simulink model "SecRwLtStCalib"  (R2024b)
settings: Solver=FixedStepDiscrete  StartTime=0.0  StopTime=10.0  FixedStep=0.01  RelTol=1e-3
model workspace (MAT data in the model file):
  KeSMSwAcsMd6SecRwLtStBkReclnUpwdDnwdPos1Max_Val : Simulink.Parameter (value not decoded)
  KeSMSwAcsMd6SecRwLtStBkReclnUpwdDnwdPos1Min_Val : Simulink.Parameter (value not decoded)
  KeSMSwAcsMd6SecRwLtStBkReclnUpwdDnwdPos1_Val : Simulink.Parameter (value not decoded)
  KeSMSwAcsMd6SecRwLtStBkReclnUpwdDnwdPosMax_Val : Simulink.Parameter (value not decoded)
  KeSMSwAcsMd6SecRwLtStBkReclnUpwdDnwdPosMin_Val : Simulink.Parameter (value not decoded)
  KeSMSwAcsMd6SecRwLtStBkReclnUpwdDnwdPos_Val : Simulink.Parameter (value not decoded)
symbols that are objects in the model workspace (value not decoded): KeSMSwAcsMd6SecRwLtStBkReclnUpwdDnwdPos1_Val, KeSMSwAcsMd6SecRwLtStBkReclnUpwdDnwdPos1Max_Val, KeSMSwAcsMd6SecRwLtStBkReclnUpwdDnwdPos1Min_Val, KeSMSwAcsMd6SecRwLtStBkReclnUpwdDnwdPos_Val, KeSMSwAcsMd6SecRwLtStBkReclnUpwdDnwdPosMax_Val, KeSMSwAcsMd6SecRwLtStBkReclnUpwdDnwdPosMin_Val
undefined symbols (not defined in the file or in its folder): KeSMSw4SAcsMd21SecRwLtStBkReclnUpwdDnwdPos_Val, KeSMSw4SAcsMd21SecRwLtStBkReclnUpwdDnwdPosMax_Val, KeSMSw4SAcsMd21SecRwLtStBkReclnUpwdDnwdPosMin_Val, KeSMSw4SAcsMd21SecRwLtStFrwdBkwdPos_Val, KeSMSw4SAcsMd21SecRwLtStFrwdBkwdPosMax_Val, KeSMSw4SAcsMd21SecRwLtStFrwdBkwdPosMin_Val, KeSMSw4SAcsMd21SecRwLtStHdrstFrwdBkwdPos_Val, KeSMSw4SAcsMd21SecRwLtStHdrstFrwdBkwdPosMax_Val, KeSMSw4SAcsMd21SecRwLtStHdrstFrwdBkwdPosMin_Val, KeSMSw4SAcsMd21SecRwLtStHdrstUpwdDnwdPos_Val, KeSMSw4SAcsMd21SecRwLtStHdrstUpwdDnwdPosMax_Val, KeSMSw4SAcsMd21SecRwLtStHdrstUpwdDnwdPosMin_Val, KeSMSw4SAcsMd22SecRwLtStBkReclnUpwdDnwdPos1_Val, KeSMSw4SAcsMd22SecRwLtStBkReclnUpwdDnwdPos2_Val, KeSMSw4SAcsMd22SecRwLtStBkReclnUpwdDnwdPos2Max_Val, KeSMSw4SAcsMd22SecRwLtStBkReclnUpwdDnwdPos2Min_Val, KeSMSw4SAcsMd22SecRwLtStBkReclnUpwdDnwdPosMax_Val, KeSMSw4SAcsMd22SecRwLtStBkReclnUpwdDnwdPosMin_Val, KeSMSw4SAcsMd22SecRwLtStFrwdBkwdPos_Val, KeSMSw4SAcsMd22SecRwLtStFrwdBkwdPosMax_Val, KeSMSw4SAcsMd22SecRwLtStFrwdBkwdPosMin_Val, KeSMSw4SAcsMd22SecRwLtStFtrstUpwdDnwdPos_Val, KeSMSw4SAcsMd22SecRwLtStFtrstUpwdDnwdPosMax_Val, KeSMSw4SAcsMd22SecRwLtStFtrstUpwdDnwdPosMin_Val, KeSMSw4SAcsMd22SecRwLtStHdrstFrwdBkwdPos_Val, KeSMSw4SAcsMd22SecRwLtStHdrstFrwdBkwdPosMax_Val, KeSMSw4SAcsMd22SecRwLtStHdrstFrwdBkwdPosMin_Val, KeSMSw4SAcsMd22SecRwLtStHdrstUpwdDnwdPos_Val, KeSMSw4SAcsMd22SecRwLtStHdrstUpwdDnwdPosMax_Val, KeSMSw4SAcsMd22SecRwLtStHdrstUpwdDnwdPosMin_Val, KeSMSw4SAcsMd22SecRwLtStLegrstOtwdInwdPos_Val, KeSMSw4SAcsMd22SecRwLtStLegrstOtwdInwdPosMax_Val, KeSMSw4SAcsMd22SecRwLtStLegrstOtwdInwdPosMin_Val, KeSMSw4SAcsMd22SecRwLtStLegrstUpwdDnwdPos_Val, KeSMSw4SAcsMd22SecRwLtStLegrstUpwdDnwdPosMax_Val, KeSMSw4SAcsMd22SecRwLtStLegrstUpwdDnwdPosMin_Val, KeSMSw4SAcsMd25SecRwLtStBkReclnUpwdDnwdPos_Val, KeSMSw4SAcsMd25SecRwLtStBkReclnUpwdDnwdPosMax_Val, KeSMSw4SAcsMd25SecRwLtStBkReclnUpwdDnwdPosMin_Val, KeSMSw4SAcsMd25SecRwLtStFrwdBkwdPos_Val, KeSMSw4SAcsMd25SecRwLtStFrwdBkwdPosMax_Val, KeSMSw4SAcsMd25SecRwLtStFrwdBkwdPosMin_Val, KeSMSw4SAcsMd25SecRwLtStHdrstFrwdBkwdPos_Val, KeSMSw4SAcsMd25SecRwLtStHdrstFrwdBkwdPosMax_Val, KeSMSw4SAcsMd25SecRwLtStHdrstFrwdBkwdPosMin_Val, KeSMSw4SAcsMd25SecRwLtStHdrstUpwdDnwdPos_Val, KeSMSw4SAcsMd25SecRwLtStHdrstUpwdDnwdPosMax_Val, KeSMSw4SAcsMd25SecRwLtStHdrstUpwdDnwdPosMin_Val, KeSMSw4SAcsMd26SecRwLtStBkReclnUpwdDnwdPos_Val, KeSMSw4SAcsMd26SecRwLtStBkReclnUpwdDnwdPosMax_Val, KeSMSw4SAcsMd26SecRwLtStBkReclnUpwdDnwdPosMin_Val, KeSMSw4SAcsMd26SecRwLtStFrwdBkwdPos_Val, KeSMSw4SAcsMd26SecRwLtStFrwdBkwdPosMax_Val, KeSMSw4SAcsMd26SecRwLtStFrwdBkwdPosMin_Val, KeSMSw4SAcsMd26SecRwLtStFtrstUpwdDnwdPos_Val, KeSMSw4SAcsMd26SecRwLtStFtrstUpwdDnwdPosMax_Val, KeSMSw4SAcsMd26SecRwLtStFtrstUpwdDnwdPosMin_Val, KeSMSw4SAcsMd26SecRwLtStHdrstFrwdBkwdPos_Val, KeSMSw4SAcsMd26SecRwLtStHdrstFrwdBkwdPosMax_Val, KeSMSw4SAcsMd26SecRwLtStHdrstFrwdBkwdPosMin_Val ... (+496)
libraries: TrgtPosSelcLib x61, StIsPosChkLib x1, simulink x1
(part 7 of 8)

== system SecRwLtStCalib/SecRwLtStLgrstInwdOtwdTrgtPosSelc_1_Cal_sys/Subsystem2/Subsystem ==
  note: 2023.8.1 V2.0.0 CR401790 增加模式21-26
  StNumFlg_Is6s_read : Inport
  Enable : EnablePort
  Constant : Constant  Value=4095  OutDataTypeStr=uint16
  Constant1 : Constant  Value=4095  OutDataTypeStr=uint16
  Constant2 : Constant  Value=4095  OutDataTypeStr=uint16
  Data Type Conversion{,1..6} (7 alike) : DataTypeConversion  SaturateOnIntegerOverflow=off  RndMeth=Floor
  PA_KeSMSw4SAcsMd22SecRwLtStLegrstOtwdInwdPosMax_Val : Constant  Value=KeSMSw4SAcsMd22SecRwLtStLegrstOtwdInwdPosMax_Val
  PA_KeSMSw4SAcsMd22SecRwLtStLegrstOtwdInwdPosMin_Val : Constant  Value=KeSMSw4SAcsMd22SecRwLtStLegrstOtwdInwdPosMin_Val
  PA_KeSMSw4SAcsMd22SecRwLtStLegrstOtwdInwdPos_Val : Constant  Value=KeSMSw4SAcsMd22SecRwLtStLegrstOtwdInwdPos_Val
  PA_KeSMSw4SAcsMd26SecRwLtStLegrstOtwdInwdPosMax_Val : Constant  Value=KeSMSw4SAcsMd26SecRwLtStLegrstOtwdInwdPosMax_Val
  PA_KeSMSw4SAcsMd26SecRwLtStLegrstOtwdInwdPosMin_Val : Constant  Value=KeSMSw4SAcsMd26SecRwLtStLegrstOtwdInwdPosMin_Val
  PA_KeSMSw4SAcsMd26SecRwLtStLegrstOtwdInwdPos_Val : Constant  Value=KeSMSw4SAcsMd26SecRwLtStLegrstOtwdInwdPos_Val
  PA_KeSMSw4SLegrstCloseMdSecRwLtStLgrstOtwdInwdPosMax_Val : Constant  Value=KeSMSw4SLegrstCloseMdSecRwLtStLgrstOtwdInwdPosMax_Val
  PA_KeSMSw4SLegrstCloseMdSecRwLtStLgrstOtwdInwdPosMin_Val : Constant  Value=KeSMSw4SLegrstCloseMdSecRwLtStLgrstOtwdInwdPosMin_Val
  PA_KeSMSw4SLegrstCloseMdSecRwLtStLgrstOtwdInwdPos_Val : Constant  Value=KeSMSw4SLegrstCloseMdSecRwLtStLgrstOtwdInwdPos_Val
  PA_KeSMSw4SLegrstOpenMdSecRwLtStLgrstOtwdInwdPosMax_Val : Constant  Value=KeSMSw4SLegrstOpenMdSecRwLtStLgrstOtwdInwdPosMax_Val
  PA_KeSMSw4SLegrstOpenMdSecRwLtStLgrstOtwdInwdPosMin_Val : Constant  Value=KeSMSw4SLegrstOpenMdSecRwLtStLgrstOtwdInwdPosMin_Val
  PA_KeSMSw4SLegrstOpenMdSecRwLtStLgrstOtwdInwdPos_Val : Constant  Value=KeSMSw4SLegrstOpenMdSecRwLtStLgrstOtwdInwdPos_Val
  PA_KeSMSw6SAcsMd56SecRwLtStLgrstInwdOtwdPosMax_Val : Constant  Value=KeSMSw6SAcsMd56SecRwLtStLgrstInwdOtwdPosMax_Val
  PA_KeSMSw6SAcsMd56SecRwLtStLgrstInwdOtwdPosMin_Val : Constant  Value=KeSMSw6SAcsMd56SecRwLtStLgrstInwdOtwdPosMin_Val
  PA_KeSMSw6SAcsMd56SecRwLtStLgrstInwdOtwdPos_Val : Constant  Value=KeSMSw6SAcsMd56SecRwLtStLgrstInwdOtwdPos_Val
  PA_KeSMSw6sAcsEntrySecRwLtStLgrstInwdOtwdPosMax_Val : Constant  Value=KeSMSw6sAcsEntrySecRwLtStLgrstInwdOtwdPosMax_Val
  PA_KeSMSw6sAcsEntrySecRwLtStLgrstInwdOtwdPosMin_Val : Constant  Value=KeSMSw6sAcsEntrySecRwLtStLgrstInwdOtwdPosMin_Val
  PA_KeSMSw6sAcsEntrySecRwLtStLgrstInwdOtwdPos_Val : Constant  Value=KeSMSw6sAcsEntrySecRwLtStLgrstInwdOtwdPos_Val
  PA_KeSMSwAcsEntrySecRwLtStLgrstInwdOtwdPosMax_Val : Constant  Value=KeSMSwAcsEntrySecRwLtStLgrstInwdOtwdPosMax_Val
  PA_KeSMSwAcsEntrySecRwLtStLgrstInwdOtwdPosMin_Val : Constant  Value=KeSMSwAcsEntrySecRwLtStLgrstInwdOtwdPosMin_Val
  PA_KeSMSwAcsEntrySecRwLtStLgrstInwdOtwdPos_Val : Constant  Value=KeSMSwAcsEntrySecRwLtStLgrstInwdOtwdPos_Val
  PA_KeSMSwAcsMd56SecRwLtStLgrstInwdOtwdPosMax_Val : Constant  Value=KeSMSwAcsMd56SecRwLtStLgrstInwdOtwdPosMax_Val
  PA_KeSMSwAcsMd56SecRwLtStLgrstInwdOtwdPosMin_Val : Constant  Value=KeSMSwAcsMd56SecRwLtStLgrstInwdOtwdPosMin_Val
  PA_KeSMSwAcsMd56SecRwLtStLgrstInwdOtwdPos_Val : Constant  Value=KeSMSwAcsMd56SecRwLtStLgrstInwdOtwdPos_Val
  PA_KeSMSwAcsMd8SecRwLtStLgrstInwdOtwdPosMax_Val : Constant  Value=KeSMSwAcsMd8SecRwLtStLgrstInwdOtwdPosMax_Val
  PA_KeSMSwAcsMd8SecRwLtStLgrstInwdOtwdPosMin_Val : Constant  Value=KeSMSwAcsMd8SecRwLtStLgrstInwdOtwdPosMin_Val
  PA_KeSMSwAcsMd8SecRwLtStLgrstInwdOtwdPos_Val : Constant  Value=KeSMSwAcsMd8SecRwLtStLgrstInwdOtwdPos_Val
  TrgtPosSelcNo4sMd : TrgtPosSelcLib/TrgtPosSelcNo4sMd  SystemSampleTime=-1  VariantActivationTime=update diagram  AllowFlexibleInterface=on  Latency=0  AutoFrameSizeCalculation=off
  TrgtPosSelcNo4sMd1 : TrgtPosSelcLib/TrgtPosSelcNo4sMd  SystemSampleTime=-1  VariantActivationTime=update diagram  AllowFlexibleInterface=on  Latency=0  AutoFrameSizeCalculation=off
  TrgtPosSelcNo4sMd2 : TrgtPosSelcLib/TrgtPosSelcNo4sMd  SystemSampleTime=-1  VariantActivationTime=update diagram  AllowFlexibleInterface=on  Latency=0  AutoFrameSizeCalculation=off
  TrgtPosSelcOnly4sMd{,1..3} (4 alike) : TrgtPosSelcLib/TrgtPosSelcOnly4sMd  SystemSampleTime=-1  VariantActivationTime=update diagram  AllowFlexibleInterface=on  Latency=0  AutoFrameSizeCalculation=off
  LgrstCloseLR2LLgrstInwdOtwdTrgtPosCalib_TrgtPosArray_write : Outport  VectorParamsAs1DForOutWhenUnconnected=off
  LgrstOpen4sLR2LLgrstInwdOtwdTrgtPosCalib_TrgtPosArray_write : Outport  Port=2  VectorParamsAs1DForOutWhenUnconnected=off
  KeSMSw4SAcsMd22LgrstInwdOtwdTrgtPosCalib_TrgtPosArray_write : Outport  Port=3  VectorParamsAs1DForOutWhenUnconnected=off
      settings: EnsureOutportIsVirtual=on
  KeSMSw4SAcsMd26LgrstInwdOtwdTrgtPosCalib_TrgtPosArray_write : Outport  Port=4  VectorParamsAs1DForOutWhenUnconnected=off
      settings: EnsureOutportIsVirtual=on
  KeSMSwEZEEntryLgrstInwdOtwdTrgtPosCalib_TrgtPosArray_write : Outport  Port=5  VectorParamsAs1DForOutWhenUnconnected=off
      settings: EnsureOutportIsVirtual=on
  Md56LgrstInwdOtwdTrgtPosCalib_TrgtPosArray_write : Outport  Port=6  VectorParamsAs1DForOutWhenUnconnected=off
      settings: EnsureOutportIsVirtual=on
  Md8R2LLgrstInwdOtwdTrgtPosCalib_TrgtPosArray_write : Outport  Port=7  VectorParamsAs1DForOutWhenUnconnected=off
      settings: EnsureOutportIsVirtual=on
  wires:
  PA_KeSMSw4SLegrstCloseMdSecRwLtStLgrstOtwdInwdPos_Val/1 -> TrgtPosSelcOnly4sMd/1
  TrgtPosSelcOnly4sMd1/1 -> Data Type Conversion1/1
  TrgtPosSelcOnly4sMd/1 -> Data Type Conversion/1
  PA_KeSMSw4SLegrstOpenMdSecRwLtStLgrstOtwdInwdPosMin_Val/1 -> TrgtPosSelcOnly4sMd1/3
  PA_KeSMSw4SLegrstOpenMdSecRwLtStLgrstOtwdInwdPosMax_Val/1 -> TrgtPosSelcOnly4sMd1/2
  PA_KeSMSw4SLegrstCloseMdSecRwLtStLgrstOtwdInwdPosMin_Val/1 -> TrgtPosSelcOnly4sMd/3
  PA_KeSMSw4SLegrstOpenMdSecRwLtStLgrstOtwdInwdPos_Val/1 -> TrgtPosSelcOnly4sMd1/1
  PA_KeSMSw4SLegrstCloseMdSecRwLtStLgrstOtwdInwdPosMax_Val/1 -> TrgtPosSelcOnly4sMd/2
  TrgtPosSelcOnly4sMd2/1 -> Data Type Conversion2/1
  TrgtPosSelcOnly4sMd3/1 -> Data Type Conversion3/1
  PA_KeSMSw4SAcsMd22SecRwLtStLegrstOtwdInwdPosMax_Val/1 -> TrgtPosSelcOnly4sMd2/2
  PA_KeSMSw4SAcsMd22SecRwLtStLegrstOtwdInwdPosMin_Val/1 -> TrgtPosSelcOnly4sMd2/3
  PA_KeSMSw4SAcsMd22SecRwLtStLegrstOtwdInwdPos_Val/1 -> TrgtPosSelcOnly4sMd2/1
  PA_KeSMSw4SAcsMd26SecRwLtStLegrstOtwdInwdPosMax_Val/1 -> TrgtPosSelcOnly4sMd3/2
  PA_KeSMSw4SAcsMd26SecRwLtStLegrstOtwdInwdPosMin_Val/1 -> TrgtPosSelcOnly4sMd3/3
  PA_KeSMSw4SAcsMd26SecRwLtStLegrstOtwdInwdPos_Val/1 -> TrgtPosSelcOnly4sMd3/1
  Data Type Conversion/1 -> LgrstCloseLR2LLgrstInwdOtwdTrgtPosCalib_TrgtPosArray_write/1
  Data Type Conversion1/1 -> LgrstOpen4sLR2LLgrstInwdOtwdTrgtPosCalib_TrgtPosArray_write/1
  Data Type Conversion2/1 -> KeSMSw4SAcsMd22LgrstInwdOtwdTrgtPosCalib_TrgtPosArray_write/1
  Data Type Conversion3/1 -> KeSMSw4SAcsMd26LgrstInwdOtwdTrgtPosCalib_TrgtPosArray_write/1
  Data Type Conversion4/1 -> KeSMSwEZEEntryLgrstInwdOtwdTrgtPosCalib_TrgtPosArray_write/1
  TrgtPosSelcNo4sMd/1 -> Data Type Conversion4/1
  StNumFlg_Is6s_read/1 -> [Is6s], TrgtPosSelcNo4sMd/1
  PA_KeSMSw6sAcsEntrySecRwLtStLgrstInwdOtwdPos_Val/1 -> TrgtPosSelcNo4sMd/2
  PA_KeSMSw6sAcsEntrySecRwLtStLgrstInwdOtwdPosMax_Val/1 -> TrgtPosSelcNo4sMd/3
  PA_KeSMSw6sAcsEntrySecRwLtStLgrstInwdOtwdPosMin_Val/1 -> TrgtPosSelcNo4sMd/4
  PA_KeSMSwAcsEntrySecRwLtStLgrstInwdOtwdPos_Val/1 -> TrgtPosSelcNo4sMd/5
  PA_KeSMSwAcsEntrySecRwLtStLgrstInwdOtwdPosMax_Val/1 -> TrgtPosSelcNo4sMd/6
  PA_KeSMSwAcsEntrySecRwLtStLgrstInwdOtwdPosMin_Val/1 -> TrgtPosSelcNo4sMd/7
  [Is6s] -> TrgtPosSelcNo4sMd1/1
  PA_KeSMSw6SAcsMd56SecRwLtStLgrstInwdOtwdPos_Val/1 -> TrgtPosSelcNo4sMd1/2
  PA_KeSMSw6SAcsMd56SecRwLtStLgrstInwdOtwdPosMax_Val/1 -> TrgtPosSelcNo4sMd1/3
  PA_KeSMSw6SAcsMd56SecRwLtStLgrstInwdOtwdPosMin_Val/1 -> TrgtPosSelcNo4sMd1/4
  PA_KeSMSwAcsMd56SecRwLtStLgrstInwdOtwdPos_Val/1 -> TrgtPosSelcNo4sMd1/5
  PA_KeSMSwAcsMd56SecRwLtStLgrstInwdOtwdPosMin_Val/1 -> TrgtPosSelcNo4sMd1/7
  PA_KeSMSwAcsMd56SecRwLtStLgrstInwdOtwdPosMax_Val/1 -> TrgtPosSelcNo4sMd1/6
  TrgtPosSelcNo4sMd1/1 -> Data Type Conversion5/1
  Data Type Conversion5/1 -> Md56LgrstInwdOtwdTrgtPosCalib_TrgtPosArray_write/1
  PA_KeSMSwAcsMd8SecRwLtStLgrstInwdOtwdPosMin_Val/1 -> TrgtPosSelcNo4sMd2/7
  Constant/1 -> TrgtPosSelcNo4sMd2/2
  PA_KeSMSwAcsMd8SecRwLtStLgrstInwdOtwdPosMax_Val/1 -> TrgtPosSelcNo4sMd2/6
  Constant1/1 -> TrgtPosSelcNo4sMd2/3
  Constant2/1 -> TrgtPosSelcNo4sMd2/4
  [Is6s] -> TrgtPosSelcNo4sMd2/1
  TrgtPosSelcNo4sMd2/1 -> Data Type Conversion6/1
  PA_KeSMSwAcsMd8SecRwLtStLgrstInwdOtwdPos_Val/1 -> TrgtPosSelcNo4sMd2/5
  Data Type Conversion6/1 -> Md8R2LLgrstInwdOtwdTrgtPosCalib_TrgtPosArray_write/1

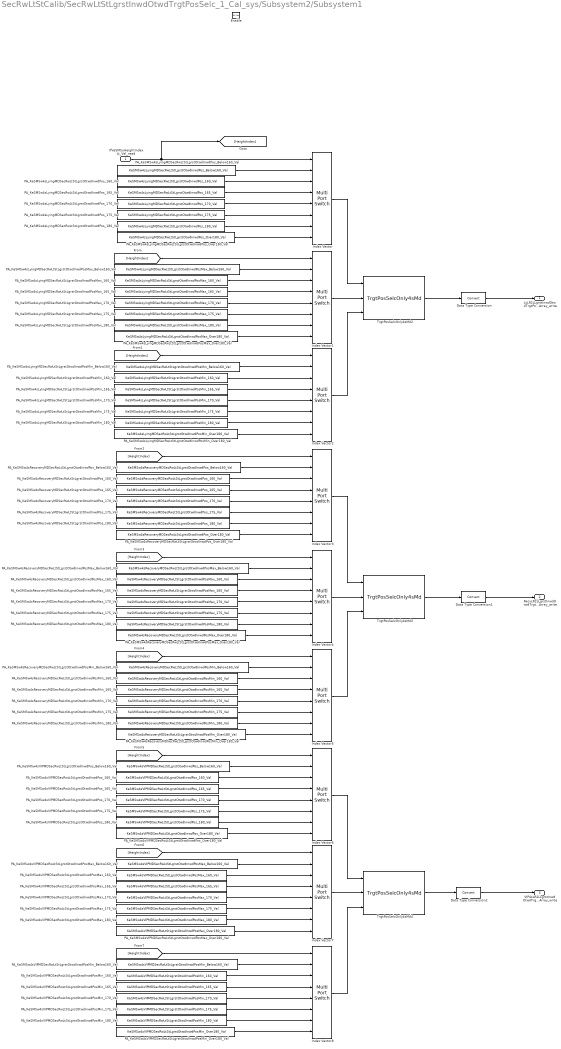
== system SecRwLtStCalib/SecRwLtStLgrstInwdOtwdTrgtPosSelc_1_Cal_sys/Subsystem2/Subsystem1 ==
  IfVeSMSuHeightIndexLt_Val_read : Inport
  Enable : EnablePort
  Data Type Conversion : DataTypeConversion  SaturateOnIntegerOverflow=off  RndMeth=Floor
  Data Type Conversion1 : DataTypeConversion  SaturateOnIntegerOverflow=off  RndMeth=Floor
  Data Type Conversion2 : DataTypeConversion  SaturateOnIntegerOverflow=off  RndMeth=Floor
  Index Vector{,1..8} (9 alike) : MultiPortSwitch  DataPortOrder=Zero-based contiguous  Inputs=7  zeroidx=on  SaturateOnIntegerOverflow=off  InputSameDT=off
  PA_KeSMSw4sLyingMDSecRwLtStLgrstOtwdInwdPosMax_160_Val : Constant  Value=KeSMSw4sLyingMDSecRwLtStLgrstOtwdInwdPosMax_160_Val
  PA_KeSMSw4sLyingMDSecRwLtStLgrstOtwdInwdPosMax_165_Val : Constant  Value=KeSMSw4sLyingMDSecRwLtStLgrstOtwdInwdPosMax_165_Val
  PA_KeSMSw4sLyingMDSecRwLtStLgrstOtwdInwdPosMax_170_Val : Constant  Value=KeSMSw4sLyingMDSecRwLtStLgrstOtwdInwdPosMax_170_Val
  PA_KeSMSw4sLyingMDSecRwLtStLgrstOtwdInwdPosMax_175_Val : Constant  Value=KeSMSw4sLyingMDSecRwLtStLgrstOtwdInwdPosMax_175_Val
  PA_KeSMSw4sLyingMDSecRwLtStLgrstOtwdInwdPosMax_180_Val : Constant  Value=KeSMSw4sLyingMDSecRwLtStLgrstOtwdInwdPosMax_180_Val
  PA_KeSMSw4sLyingMDSecRwLtStLgrstOtwdInwdPosMax_Below160_Val : Constant  Value=KeSMSw4sLyingMDSecRwLtStLgrstOtwdInwdPosMax_Below160_Val
  PA_KeSMSw4sLyingMDSecRwLtStLgrstOtwdInwdPosMax_Over180_Val : Constant  Value=KeSMSw4sLyingMDSecRwLtStLgrstOtwdInwdPosMax_Over180_Val
  PA_KeSMSw4sLyingMDSecRwLtStLgrstOtwdInwdPosMin_160_Val : Constant  Value=KeSMSw4sLyingMDSecRwLtStLgrstOtwdInwdPosMin_160_Val
  PA_KeSMSw4sLyingMDSecRwLtStLgrstOtwdInwdPosMin_165_Val : Constant  Value=KeSMSw4sLyingMDSecRwLtStLgrstOtwdInwdPosMin_165_Val
  PA_KeSMSw4sLyingMDSecRwLtStLgrstOtwdInwdPosMin_170_Val : Constant  Value=KeSMSw4sLyingMDSecRwLtStLgrstOtwdInwdPosMin_170_Val
  PA_KeSMSw4sLyingMDSecRwLtStLgrstOtwdInwdPosMin_175_Val : Constant  Value=KeSMSw4sLyingMDSecRwLtStLgrstOtwdInwdPosMin_175_Val
  PA_KeSMSw4sLyingMDSecRwLtStLgrstOtwdInwdPosMin_180_Val : Constant  Value=KeSMSw4sLyingMDSecRwLtStLgrstOtwdInwdPosMin_180_Val
  PA_KeSMSw4sLyingMDSecRwLtStLgrstOtwdInwdPosMin_Below160_Val : Constant  Value=KeSMSw4sLyingMDSecRwLtStLgrstOtwdInwdPosMin_Below160_Val
  PA_KeSMSw4sLyingMDSecRwLtStLgrstOtwdInwdPosMin_Over180_Val : Constant  Value=KeSMSw4sLyingMDSecRwLtStLgrstOtwdInwdPosMin_Over180_Val
  PA_KeSMSw4sLyingMDSecRwLtStLgrstOtwdInwdPos_160_Val : Constant  Value=KeSMSw4sLyingMDSecRwLtStLgrstOtwdInwdPos_160_Val
  PA_KeSMSw4sLyingMDSecRwLtStLgrstOtwdInwdPos_165_Val : Constant  Value=KeSMSw4sLyingMDSecRwLtStLgrstOtwdInwdPos_165_Val
  PA_KeSMSw4sLyingMDSecRwLtStLgrstOtwdInwdPos_170_Val : Constant  Value=KeSMSw4sLyingMDSecRwLtStLgrstOtwdInwdPos_170_Val
  PA_KeSMSw4sLyingMDSecRwLtStLgrstOtwdInwdPos_175_Val : Constant  Value=KeSMSw4sLyingMDSecRwLtStLgrstOtwdInwdPos_175_Val
  PA_KeSMSw4sLyingMDSecRwLtStLgrstOtwdInwdPos_180_Val : Constant  Value=KeSMSw4sLyingMDSecRwLtStLgrstOtwdInwdPos_180_Val
  PA_KeSMSw4sLyingMDSecRwLtStLgrstOtwdInwdPos_Below160_Val : Constant  Value=KeSMSw4sLyingMDSecRwLtStLgrstOtwdInwdPos_Below160_Val
  PA_KeSMSw4sLyingMDSecRwLtStLgrstOtwdInwdPos_Over180_Val : Constant  Value=KeSMSw4sLyingMDSecRwLtStLgrstOtwdInwdPos_Over180_Val
  PA_KeSMSw4sRecoveryMDSecRwLtStLgrstOtwdInwdPosMax_160_Val : Constant  Value=KeSMSw4sRecoveryMDSecRwLtStLgrstOtwdInwdPosMax_160_Val
  PA_KeSMSw4sRecoveryMDSecRwLtStLgrstOtwdInwdPosMax_165_Val : Constant  Value=KeSMSw4sRecoveryMDSecRwLtStLgrstOtwdInwdPosMax_165_Val
  PA_KeSMSw4sRecoveryMDSecRwLtStLgrstOtwdInwdPosMax_170_Val : Constant  Value=KeSMSw4sRecoveryMDSecRwLtStLgrstOtwdInwdPosMax_170_Val
  PA_KeSMSw4sRecoveryMDSecRwLtStLgrstOtwdInwdPosMax_175_Val : Constant  Value=KeSMSw4sRecoveryMDSecRwLtStLgrstOtwdInwdPosMax_175_Val
  PA_KeSMSw4sRecoveryMDSecRwLtStLgrstOtwdInwdPosMax_180_Val : Constant  Value=KeSMSw4sRecoveryMDSecRwLtStLgrstOtwdInwdPosMax_180_Val
  PA_KeSMSw4sRecoveryMDSecRwLtStLgrstOtwdInwdPosMax_Below160_Val : Constant  Value=KeSMSw4sRecoveryMDSecRwLtStLgrstOtwdInwdPosMax_Below160_Val
  PA_KeSMSw4sRecoveryMDSecRwLtStLgrstOtwdInwdPosMax_Over180_Val : Constant  Value=KeSMSw4sRecoveryMDSecRwLtStLgrstOtwdInwdPosMax_Over180_Val
  PA_KeSMSw4sRecoveryMDSecRwLtStLgrstOtwdInwdPosMin_160_Val : Constant  Value=KeSMSw4sRecoveryMDSecRwLtStLgrstOtwdInwdPosMin_160_Val
  PA_KeSMSw4sRecoveryMDSecRwLtStLgrstOtwdInwdPosMin_165_Val : Constant  Value=KeSMSw4sRecoveryMDSecRwLtStLgrstOtwdInwdPosMin_165_Val
  PA_KeSMSw4sRecoveryMDSecRwLtStLgrstOtwdInwdPosMin_170_Val : Constant  Value=KeSMSw4sRecoveryMDSecRwLtStLgrstOtwdInwdPosMin_170_Val
  PA_KeSMSw4sRecoveryMDSecRwLtStLgrstOtwdInwdPosMin_175_Val : Constant  Value=KeSMSw4sRecoveryMDSecRwLtStLgrstOtwdInwdPosMin_175_Val
  PA_KeSMSw4sRecoveryMDSecRwLtStLgrstOtwdInwdPosMin_180_Val : Constant  Value=KeSMSw4sRecoveryMDSecRwLtStLgrstOtwdInwdPosMin_180_Val
  PA_KeSMSw4sRecoveryMDSecRwLtStLgrstOtwdInwdPosMin_Below160_Val : Constant  Value=KeSMSw4sRecoveryMDSecRwLtStLgrstOtwdInwdPosMin_Below160_Val
  PA_KeSMSw4sRecoveryMDSecRwLtStLgrstOtwdInwdPosMin_Over180_Val : Constant  Value=KeSMSw4sRecoveryMDSecRwLtStLgrstOtwdInwdPosMin_Over180_Val
  PA_KeSMSw4sRecoveryMDSecRwLtStLgrstOtwdInwdPos_160_Val : Constant  Value=KeSMSw4sRecoveryMDSecRwLtStLgrstOtwdInwdPos_160_Val
  PA_KeSMSw4sRecoveryMDSecRwLtStLgrstOtwdInwdPos_165_Val : Constant  Value=KeSMSw4sRecoveryMDSecRwLtStLgrstOtwdInwdPos_165_Val
  PA_KeSMSw4sRecoveryMDSecRwLtStLgrstOtwdInwdPos_170_Val : Constant  Value=KeSMSw4sRecoveryMDSecRwLtStLgrstOtwdInwdPos_170_Val
  PA_KeSMSw4sRecoveryMDSecRwLtStLgrstOtwdInwdPos_175_Val : Constant  Value=KeSMSw4sRecoveryMDSecRwLtStLgrstOtwdInwdPos_175_Val
  PA_KeSMSw4sRecoveryMDSecRwLtStLgrstOtwdInwdPos_180_Val : Constant  Value=KeSMSw4sRecoveryMDSecRwLtStLgrstOtwdInwdPos_180_Val
  PA_KeSMSw4sRecoveryMDSecRwLtStLgrstOtwdInwdPos_Below160_Val : Constant  Value=KeSMSw4sRecoveryMDSecRwLtStLgrstOtwdInwdPos_Below160_Val
  PA_KeSMSw4sRecoveryMDSecRwLtStLgrstOtwdInwdPos_Over180_Val : Constant  Value=KeSMSw4sRecoveryMDSecRwLtStLgrstOtwdInwdPos_Over180_Val
  PA_KeSMSw4sVIPMDSecRwLtStLgrstOtwdInwdPosMax_160_Val : Constant  Value=KeSMSw4sVIPMDSecRwLtStLgrstOtwdInwdPosMax_160_Val
  PA_KeSMSw4sVIPMDSecRwLtStLgrstOtwdInwdPosMax_165_Val : Constant  Value=KeSMSw4sVIPMDSecRwLtStLgrstOtwdInwdPosMax_165_Val
  PA_KeSMSw4sVIPMDSecRwLtStLgrstOtwdInwdPosMax_170_Val : Constant  Value=KeSMSw4sVIPMDSecRwLtStLgrstOtwdInwdPosMax_170_Val
  PA_KeSMSw4sVIPMDSecRwLtStLgrstOtwdInwdPosMax_175_Val : Constant  Value=KeSMSw4sVIPMDSecRwLtStLgrstOtwdInwdPosMax_175_Val
  PA_KeSMSw4sVIPMDSecRwLtStLgrstOtwdInwdPosMax_180_Val : Constant  Value=KeSMSw4sVIPMDSecRwLtStLgrstOtwdInwdPosMax_180_Val
  PA_KeSMSw4sVIPMDSecRwLtStLgrstOtwdInwdPosMax_Below160_Val : Constant  Value=KeSMSw4sVIPMDSecRwLtStLgrstOtwdInwdPosMax_Below160_Val
  PA_KeSMSw4sVIPMDSecRwLtStLgrstOtwdInwdPosMax_Over180_Val : Constant  Value=KeSMSw4sVIPMDSecRwLtStLgrstOtwdInwdPosMax_Over180_Val
  PA_KeSMSw4sVIPMDSecRwLtStLgrstOtwdInwdPosMin_160_Val : Constant  Value=KeSMSw4sVIPMDSecRwLtStLgrstOtwdInwdPosMin_160_Val
  PA_KeSMSw4sVIPMDSecRwLtStLgrstOtwdInwdPosMin_165_Val : Constant  Value=KeSMSw4sVIPMDSecRwLtStLgrstOtwdInwdPosMin_165_Val
  PA_KeSMSw4sVIPMDSecRwLtStLgrstOtwdInwdPosMin_170_Val : Constant  Value=KeSMSw4sVIPMDSecRwLtStLgrstOtwdInwdPosMin_170_Val
  PA_KeSMSw4sVIPMDSecRwLtStLgrstOtwdInwdPosMin_175_Val : Constant  Value=KeSMSw4sVIPMDSecRwLtStLgrstOtwdInwdPosMin_175_Val
  PA_KeSMSw4sVIPMDSecRwLtStLgrstOtwdInwdPosMin_180_Val : Constant  Value=KeSMSw4sVIPMDSecRwLtStLgrstOtwdInwdPosMin_180_Val
  PA_KeSMSw4sVIPMDSecRwLtStLgrstOtwdInwdPosMin_Below160_Val : Constant  Value=KeSMSw4sVIPMDSecRwLtStLgrstOtwdInwdPosMin_Below160_Val
  PA_KeSMSw4sVIPMDSecRwLtStLgrstOtwdInwdPosMin_Over180_Val : Constant  Value=KeSMSw4sVIPMDSecRwLtStLgrstOtwdInwdPosMin_Over180_Val
  PA_KeSMSw4sVIPMDSecRwLtStLgrstOtwdInwdPos_160_Val : Constant  Value=KeSMSw4sVIPMDSecRwLtStLgrstOtwdInwdPos_160_Val
  PA_KeSMSw4sVIPMDSecRwLtStLgrstOtwdInwdPos_165_Val : Constant  Value=KeSMSw4sVIPMDSecRwLtStLgrstOtwdInwdPos_165_Val
  PA_KeSMSw4sVIPMDSecRwLtStLgrstOtwdInwdPos_170_Val : Constant  Value=KeSMSw4sVIPMDSecRwLtStLgrstOtwdInwdPos_170_Val
  PA_KeSMSw4sVIPMDSecRwLtStLgrstOtwdInwdPos_175_Val : Constant  Value=KeSMSw4sVIPMDSecRwLtStLgrstOtwdInwdPos_175_Val
  PA_KeSMSw4sVIPMDSecRwLtStLgrstOtwdInwdPos_180_Val : Constant  Value=KeSMSw4sVIPMDSecRwLtStLgrstOtwdInwdPos_180_Val
  PA_KeSMSw4sVIPMDSecRwLtStLgrstOtwdInwdPos_Below160_Val : Constant  Value=KeSMSw4sVIPMDSecRwLtStLgrstOtwdInwdPos_Below160_Val
  PA_KeSMSw4sVIPMDSecRwLtStLgrstOtwdInwdPos_Over180_Val : Constant  Value=KeSMSw4sVIPMDSecRwLtStLgrstOtwdInwdPos_Over180_Val
  TrgtPosSelcOnly4sMd2 : TrgtPosSelcLib/TrgtPosSelcOnly4sMd  SystemSampleTime=-1  VariantActivationTime=update diagram  AllowFlexibleInterface=on  Latency=0  AutoFrameSizeCalculation=off
  TrgtPosSelcOnly4sMd3 : TrgtPosSelcLib/TrgtPosSelcOnly4sMd  SystemSampleTime=-1  VariantActivationTime=update diagram  AllowFlexibleInterface=on  Latency=0  AutoFrameSizeCalculation=off
  TrgtPosSelcOnly4sMd4 : TrgtPosSelcLib/TrgtPosSelcOnly4sMd  SystemSampleTime=-1  VariantActivationTime=update diagram  AllowFlexibleInterface=on  Latency=0  AutoFrameSizeCalculation=off
  LyLR2LLgrstInwdOtwdTrgtPosCalib_TrgtPosArray_write : Outport  VectorParamsAs1DForOutWhenUnconnected=off
  RecvLR2LLgrstInwdOtwdTrgtPosCalib_TrgtPosArray_write : Outport  Port=2  VectorParamsAs1DForOutWhenUnconnected=off
  VIP4sLR2LLgrstInwdOtwdTrgtPosCalib_TrgtPosArray_write : Outport  Port=3  VectorParamsAs1DForOutWhenUnconnected=off
  wires:
  PA_KeSMSw4sRecoveryMDSecRwLtStLgrstOtwdInwdPos_Below160_Val/1 -> Index Vector3/2
  PA_KeSMSw4sVIPMDSecRwLtStLgrstOtwdInwdPosMax_180_Val/1 -> Index Vector7/7
  PA_KeSMSw4sLyingMDSecRwLtStLgrstOtwdInwdPos_Below160_Val/1 -> Index Vector/2
  PA_KeSMSw4sRecoveryMDSecRwLtStLgrstOtwdInwdPosMin_175_Val/1 -> Index Vector5/6
  PA_KeSMSw4sVIPMDSecRwLtStLgrstOtwdInwdPosMin_Over180_Val/1 -> Index Vector8/8
  PA_KeSMSw4sVIPMDSecRwLtStLgrstOtwdInwdPosMin_180_Val/1 -> Index Vector8/7
  IfVeSMSuHeightIndexLt_Val_read/1 -> [HeightIndex], Index Vector/1
  PA_KeSMSw4sLyingMDSecRwLtStLgrstOtwdInwdPos_170_Val/1 -> Index Vector/5
  PA_KeSMSw4sRecoveryMDSecRwLtStLgrstOtwdInwdPos_165_Val/1 -> Index Vector3/4
  PA_KeSMSw4sLyingMDSecRwLtStLgrstOtwdInwdPosMin_Below160_Val/1 -> Index Vector2/2
  PA_KeSMSw4sLyingMDSecRwLtStLgrstOtwdInwdPosMax_180_Val/1 -> Index Vector1/7
  PA_KeSMSw4sLyingMDSecRwLtStLgrstOtwdInwdPosMin_175_Val/1 -> Index Vector2/6
  PA_KeSMSw4sRecoveryMDSecRwLtStLgrstOtwdInwdPosMax_175_Val/1 -> Index Vector4/6
  PA_KeSMSw4sRecoveryMDSecRwLtStLgrstOtwdInwdPos_170_Val/1 -> Index Vector3/5
  TrgtPosSelcOnly4sMd3/1 -> Data Type Conversion1/1
  [HeightIndex] -> Index Vector1/1
  PA_KeSMSw4sVIPMDSecRwLtStLgrstOtwdInwdPos_165_Val/1 -> Index Vector6/4
  PA_KeSMSw4sLyingMDSecRwLtStLgrstOtwdInwdPos_180_Val/1 -> Index Vector/7
  PA_KeSMSw4sVIPMDSecRwLtStLgrstOtwdInwdPos_175_Val/1 -> Index Vector6/6
  PA_KeSMSw4sLyingMDSecRwLtStLgrstOtwdInwdPosMax_Over180_Val/1 -> Index Vector1/8
  PA_KeSMSw4sRecoveryMDSecRwLtStLgrstOtwdInwdPosMax_180_Val/1 -> Index Vector4/7
  [HeightIndex] -> Index Vector8/1
  PA_KeSMSw4sLyingMDSecRwLtStLgrstOtwdInwdPosMin_180_Val/1 -> Index Vector2/7
  PA_KeSMSw4sLyingMDSecRwLtStLgrstOtwdInwdPosMax_170_Val/1 -> Index Vector1/5
  PA_KeSMSw4sLyingMDSecRwLtStLgrstOtwdInwdPosMax_Below160_Val/1 -> Index Vector1/2
  PA_KeSMSw4sVIPMDSecRwLtStLgrstOtwdInwdPosMax_Below160_Val/1 -> Index Vector7/2
  PA_KeSMSw4sLyingMDSecRwLtStLgrstOtwdInwdPos_175_Val/1 -> Index Vector/6
  TrgtPosSelcOnly4sMd2/1 -> Data Type Conversion/1
  [HeightIndex] -> Index Vector2/1
  [HeightIndex] -> Index Vector4/1
  PA_KeSMSw4sRecoveryMDSecRwLtStLgrstOtwdInwdPosMax_170_Val/1 -> Index Vector4/5
  PA_KeSMSw4sLyingMDSecRwLtStLgrstOtwdInwdPosMin_Over180_Val/1 -> Index Vector2/8
  PA_KeSMSw4sRecoveryMDSecRwLtStLgrstOtwdInwdPos_180_Val/1 -> Index Vector3/7
  PA_KeSMSw4sRecoveryMDSecRwLtStLgrstOtwdInwdPosMin_180_Val/1 -> Index Vector5/7
  PA_KeSMSw4sLyingMDSecRwLtStLgrstOtwdInwdPosMin_170_Val/1 -> Index Vector2/5
  [HeightIndex] -> Index Vector6/1
  PA_KeSMSw4sLyingMDSecRwLtStLgrstOtwdInwdPos_Over180_Val/1 -> Index Vector/8
  PA_KeSMSw4sVIPMDSecRwLtStLgrstOtwdInwdPosMax_Over180_Val/1 -> Index Vector7/8
  [HeightIndex] -> Index Vector7/1
  PA_KeSMSw4sVIPMDSecRwLtStLgrstOtwdInwdPos_180_Val/1 -> Index Vector6/7
  PA_KeSMSw4sRecoveryMDSecRwLtStLgrstOtwdInwdPosMin_170_Val/1 -> Index Vector5/5
  TrgtPosSelcOnly4sMd4/1 -> Data Type Conversion2/1
  [HeightIndex] -> Index Vector5/1
  PA_KeSMSw4sRecoveryMDSecRwLtStLgrstOtwdInwdPosMax_165_Val/1 -> Index Vector4/4
  PA_KeSMSw4sLyingMDSecRwLtStLgrstOtwdInwdPos_160_Val/1 -> Index Vector/3
  PA_KeSMSw4sRecoveryMDSecRwLtStLgrstOtwdInwdPos_175_Val/1 -> Index Vector3/6
  PA_KeSMSw4sVIPMDSecRwLtStLgrstOtwdInwdPosMax_165_Val/1 -> Index Vector7/4
  PA_KeSMSw4sVIPMDSecRwLtStLgrstOtwdInwdPosMin_165_Val/1 -> Index Vector8/4
  PA_KeSMSw4sLyingMDSecRwLtStLgrstOtwdInwdPosMin_160_Val/1 -> Index Vector2/3
  PA_KeSMSw4sLyingMDSecRwLtStLgrstOtwdInwdPosMin_165_Val/1 -> Index Vector2/4
  PA_KeSMSw4sRecoveryMDSecRwLtStLgrstOtwdInwdPosMax_160_Val/1 -> Index Vector4/3
  [HeightIndex] -> Index Vector3/1
  PA_KeSMSw4sRecoveryMDSecRwLtStLgrstOtwdInwdPos_Over180_Val/1 -> Index Vector3/8
  PA_KeSMSw4sLyingMDSecRwLtStLgrstOtwdInwdPosMax_165_Val/1 -> Index Vector1/4
  PA_KeSMSw4sVIPMDSecRwLtStLgrstOtwdInwdPos_160_Val/1 -> Index Vector6/3
  PA_KeSMSw4sLyingMDSecRwLtStLgrstOtwdInwdPosMax_175_Val/1 -> Index Vector1/6
  PA_KeSMSw4sRecoveryMDSecRwLtStLgrstOtwdInwdPosMin_160_Val/1 -> Index Vector5/3
  PA_KeSMSw4sVIPMDSecRwLtStLgrstOtwdInwdPos_Over180_Val/1 -> Index Vector6/8
  PA_KeSMSw4sLyingMDSecRwLtStLgrstOtwdInwdPos_165_Val/1 -> Index Vector/4
  PA_KeSMSw4sRecoveryMDSecRwLtStLgrstOtwdInwdPosMin_Below160_Val/1 -> Index Vector5/2
  PA_KeSMSw4sRecoveryMDSecRwLtStLgrstOtwdInwdPosMin_Over180_Val/1 -> Index Vector5/8
  PA_KeSMSw4sVIPMDSecRwLtStLgrstOtwdInwdPosMax_175_Val/1 -> Index Vector7/6
  PA_KeSMSw4sVIPMDSecRwLtStLgrstOtwdInwdPosMax_160_Val/1 -> Index Vector7/3
  PA_KeSMSw4sRecoveryMDSecRwLtStLgrstOtwdInwdPos_160_Val/1 -> Index Vector3/3
  PA_KeSMSw4sRecoveryMDSecRwLtStLgrstOtwdInwdPosMin_165_Val/1 -> Index Vector5/4
  PA_KeSMSw4sVIPMDSecRwLtStLgrstOtwdInwdPosMin_160_Val/1 -> Index Vector8/3
  Index Vector/1 -> TrgtPosSelcOnly4sMd2/1
  Index Vector1/1 -> TrgtPosSelcOnly4sMd2/2
  PA_KeSMSw4sVIPMDSecRwLtStLgrstOtwdInwdPos_170_Val/1 -> Index Vector6/5
  Index Vector2/1 -> TrgtPosSelcOnly4sMd2/3
  PA_KeSMSw4sRecoveryMDSecRwLtStLgrstOtwdInwdPosMax_Below160_Val/1 -> Index Vector4/2
  PA_KeSMSw4sVIPMDSecRwLtStLgrstOtwdInwdPosMin_170_Val/1 -> Index Vector8/5
  Index Vector7/1 -> TrgtPosSelcOnly4sMd4/2
  Index Vector5/1 -> TrgtPosSelcOnly4sMd3/3
  Index Vector4/1 -> TrgtPosSelcOnly4sMd3/2
  PA_KeSMSw4sVIPMDSecRwLtStLgrstOtwdInwdPos_Below160_Val/1 -> Index Vector6/2
  PA_KeSMSw4sLyingMDSecRwLtStLgrstOtwdInwdPosMax_160_Val/1 -> Index Vector1/3
  Index Vector6/1 -> TrgtPosSelcOnly4sMd4/1
  PA_KeSMSw4sVIPMDSecRwLtStLgrstOtwdInwdPosMin_Below160_Val/1 -> Index Vector8/2
  PA_KeSMSw4sRecoveryMDSecRwLtStLgrstOtwdInwdPosMax_Over180_Val/1 -> Index Vector4/8
  Index Vector8/1 -> TrgtPosSelcOnly4sMd4/3
  PA_KeSMSw4sVIPMDSecRwLtStLgrstOtwdInwdPosMax_170_Val/1 -> Index Vector7/5
  PA_KeSMSw4sVIPMDSecRwLtStLgrstOtwdInwdPosMin_175_Val/1 -> Index Vector8/6
  Index Vector3/1 -> TrgtPosSelcOnly4sMd3/1
  Data Type Conversion/1 -> LyLR2LLgrstInwdOtwdTrgtPosCalib_TrgtPosArray_write/1
  Data Type Conversion1/1 -> RecvLR2LLgrstInwdOtwdTrgtPosCalib_TrgtPosArray_write/1
  Data Type Conversion2/1 -> VIP4sLR2LLgrstInwdOtwdTrgtPosCalib_TrgtPosArray_write/1

== system SecRwLtStCalib/SecRwLtStLgrstInwdOtwdTrgtPosSelc_1_Cal_sys/Subsystem2/Subsystem2 ==
  StNumFlg_Is6s_read : Inport
  Enable : EnablePort
  Data Type Conversion1 : DataTypeConversion  SaturateOnIntegerOverflow=off  RndMeth=Floor
  PA_KeSMSw6sRecoveryMdSecRwLtStLgrstInwdOtwdPosMax_Val : Constant  Value=KeSMSw6sRecoveryMdSecRwLtStLgrstInwdOtwdPosMax_Val
  PA_KeSMSw6sRecoveryMdSecRwLtStLgrstInwdOtwdPosMin_Val : Constant  Value=KeSMSw6sRecoveryMdSecRwLtStLgrstInwdOtwdPosMin_Val
  PA_KeSMSw6sRecoveryMdSecRwLtStLgrstInwdOtwdPos_Val : Constant  Value=KeSMSw6sRecoveryMdSecRwLtStLgrstInwdOtwdPos_Val
  PA_KeSMSwRecoveryMdSecRwLtStLgrstInwdOtwdPosMax_Val : Constant  Value=KeSMSwRecoveryMdSecRwLtStLgrstInwdOtwdPosMax_Val
  PA_KeSMSwRecoveryMdSecRwLtStLgrstInwdOtwdPosMin_Val : Constant  Value=KeSMSwRecoveryMdSecRwLtStLgrstInwdOtwdPosMin_Val
  PA_KeSMSwRecoveryMdSecRwLtStLgrstInwdOtwdPos_Val : Constant  Value=KeSMSwRecoveryMdSecRwLtStLgrstInwdOtwdPos_Val
  TrgtPosSelcNo4sMd : TrgtPosSelcLib/TrgtPosSelcNo4sMd  SystemSampleTime=-1  VariantActivationTime=update diagram  AllowFlexibleInterface=on  Latency=0  AutoFrameSizeCalculation=off
  RecvLR2LLgrstInwdOtwdTrgtPosCalib_TrgtPosArray_write : Outport  VectorParamsAs1DForOutWhenUnconnected=off
  wires:
  Data Type Conversion1/1 -> RecvLR2LLgrstInwdOtwdTrgtPosCalib_TrgtPosArray_write/1
  TrgtPosSelcNo4sMd/1 -> Data Type Conversion1/1
  StNumFlg_Is6s_read/1 -> TrgtPosSelcNo4sMd/1
  PA_KeSMSw6sRecoveryMdSecRwLtStLgrstInwdOtwdPos_Val/1 -> TrgtPosSelcNo4sMd/2
  PA_KeSMSw6sRecoveryMdSecRwLtStLgrstInwdOtwdPosMax_Val/1 -> TrgtPosSelcNo4sMd/3
  PA_KeSMSw6sRecoveryMdSecRwLtStLgrstInwdOtwdPosMin_Val/1 -> TrgtPosSelcNo4sMd/4
  PA_KeSMSwRecoveryMdSecRwLtStLgrstInwdOtwdPos_Val/1 -> TrgtPosSelcNo4sMd/5
  PA_KeSMSwRecoveryMdSecRwLtStLgrstInwdOtwdPosMax_Val/1 -> TrgtPosSelcNo4sMd/6
  PA_KeSMSwRecoveryMdSecRwLtStLgrstInwdOtwdPosMin_Val/1 -> TrgtPosSelcNo4sMd/7

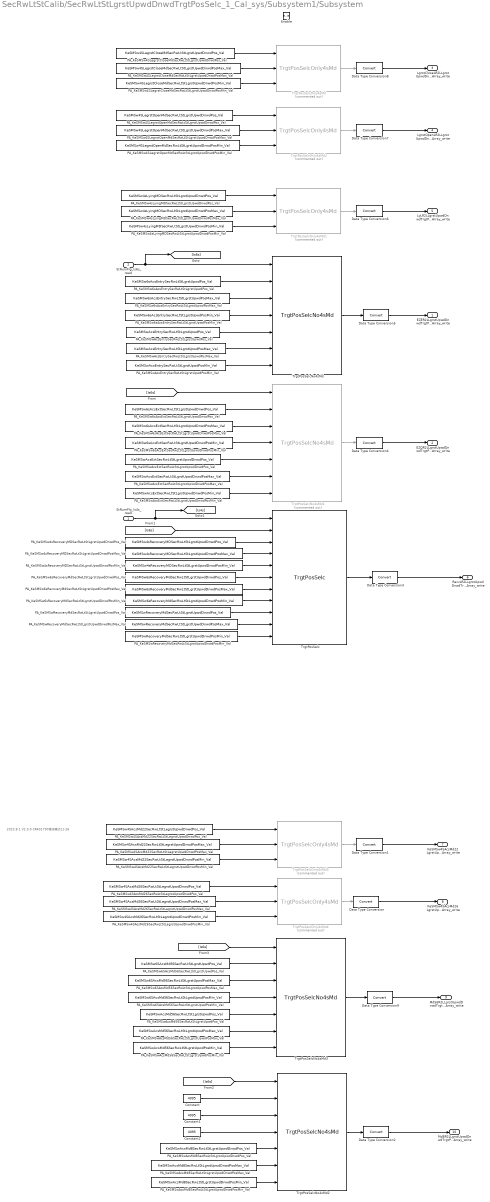
== system SecRwLtStCalib/SecRwLtStLgrstUpwdDnwdTrgtPosSelc_1_Cal_sys/Subsystem1/Subsystem ==
  note: 2023.8.1 V2.0.0 CR401790 增加模式21-26
  StNumFlg_Is4s_read : Inport
  StNumFlg_Is6s_read : Inport  Port=2
  Enable : EnablePort
  Constant : Constant  Value=4095  OutDataTypeStr=uint16
  Constant1 : Constant  Value=4095  OutDataTypeStr=uint16
  Constant2 : Constant  Value=4095  OutDataTypeStr=uint16
  Data Type Conversion{,1..9} (10 alike) : DataTypeConversion  SaturateOnIntegerOverflow=off  RndMeth=Floor
  PA_KeSMSw4SAcsMd22SecRwLtStLegrstUpwdDnwdPosMax_Val : Constant  Value=KeSMSw4SAcsMd22SecRwLtStLegrstUpwdDnwdPosMax_Val
  PA_KeSMSw4SAcsMd22SecRwLtStLegrstUpwdDnwdPosMin_Val : Constant  Value=KeSMSw4SAcsMd22SecRwLtStLegrstUpwdDnwdPosMin_Val
  PA_KeSMSw4SAcsMd22SecRwLtStLegrstUpwdDnwdPos_Val : Constant  Value=KeSMSw4SAcsMd22SecRwLtStLegrstUpwdDnwdPos_Val
  PA_KeSMSw4SAcsMd26SecRwLtStLegrstUpwdDnwdPosMax_Val : Constant  Value=KeSMSw4SAcsMd26SecRwLtStLegrstUpwdDnwdPosMax_Val
  PA_KeSMSw4SAcsMd26SecRwLtStLegrstUpwdDnwdPosMin_Val : Constant  Value=KeSMSw4SAcsMd26SecRwLtStLegrstUpwdDnwdPosMin_Val
  PA_KeSMSw4SAcsMd26SecRwLtStLegrstUpwdDnwdPos_Val : Constant  Value=KeSMSw4SAcsMd26SecRwLtStLegrstUpwdDnwdPos_Val
  PA_KeSMSw4SLegrstCloseMdSecRwLtStLgrstUpwdDnwdPosMax_Val : Constant  Value=KeSMSw4SLegrstCloseMdSecRwLtStLgrstUpwdDnwdPosMax_Val
  PA_KeSMSw4SLegrstCloseMdSecRwLtStLgrstUpwdDnwdPosMin_Val : Constant  Value=KeSMSw4SLegrstCloseMdSecRwLtStLgrstUpwdDnwdPosMin_Val
  PA_KeSMSw4SLegrstCloseMdSecRwLtStLgrstUpwdDnwdPos_Val : Constant  Value=KeSMSw4SLegrstCloseMdSecRwLtStLgrstUpwdDnwdPos_Val
  PA_KeSMSw4SLegrstOpenMdSecRwLtStLgrstUpwdDnwdPosMax_Val : Constant  Value=KeSMSw4SLegrstOpenMdSecRwLtStLgrstUpwdDnwdPosMax_Val
  PA_KeSMSw4SLegrstOpenMdSecRwLtStLgrstUpwdDnwdPosMin_Val : Constant  Value=KeSMSw4SLegrstOpenMdSecRwLtStLgrstUpwdDnwdPosMin_Val
  PA_KeSMSw4SLegrstOpenMdSecRwLtStLgrstUpwdDnwdPos_Val : Constant  Value=KeSMSw4SLegrstOpenMdSecRwLtStLgrstUpwdDnwdPos_Val
  PA_KeSMSw4sLyingMDSecRwLtStLgrstUpwdDnwdPosMax_Val : Constant  Value=KeSMSw4sLyingMDSecRwLtStLgrstUpwdDnwdPosMax_Val
  PA_KeSMSw4sLyingMDSecRwLtStLgrstUpwdDnwdPosMin_Val : Constant  Value=KeSMSw4sLyingMDSecRwLtStLgrstUpwdDnwdPosMin_Val
  PA_KeSMSw4sLyingMDSecRwLtStLgrstUpwdDnwdPos_Val : Constant  Value=KeSMSw4sLyingMDSecRwLtStLgrstUpwdDnwdPos_Val
  PA_KeSMSw4sRecoveryMDSecRwLtStLgrstUpwdDnwdPosMax_Val : Constant  Value=KeSMSw4sRecoveryMDSecRwLtStLgrstUpwdDnwdPosMax_Val
  PA_KeSMSw4sRecoveryMDSecRwLtStLgrstUpwdDnwdPosMin_Val : Constant  Value=KeSMSw4sRecoveryMDSecRwLtStLgrstUpwdDnwdPosMin_Val
  PA_KeSMSw4sRecoveryMDSecRwLtStLgrstUpwdDnwdPos_Val : Constant  Value=KeSMSw4sRecoveryMDSecRwLtStLgrstUpwdDnwdPos_Val
  PA_KeSMSw6SAcsMd56SecRwLtStLgrstUpwdPosMax_Val : Constant  Value=KeSMSw6SAcsMd56SecRwLtStLgrstUpwdPosMax_Val
  PA_KeSMSw6SAcsMd56SecRwLtStLgrstUpwdPosMin_Val : Constant  Value=KeSMSw6SAcsMd56SecRwLtStLgrstUpwdPosMin_Val
  PA_KeSMSw6SAcsMd56SecRwLtStLgrstUpwdPos_Val : Constant  Value=KeSMSw6SAcsMd56SecRwLtStLgrstUpwdPos_Val
  PA_KeSMSw6sAcsEntrySecRwLtStLgrstUpwdPosMax_Val : Constant  Value=KeSMSw6sAcsEntrySecRwLtStLgrstUpwdPosMax_Val
  PA_KeSMSw6sAcsEntrySecRwLtStLgrstUpwdPosMin_Val : Constant  Value=KeSMSw6sAcsEntrySecRwLtStLgrstUpwdPosMin_Val
  PA_KeSMSw6sAcsEntrySecRwLtStLgrstUpwdPos_Val : Constant  Value=KeSMSw6sAcsEntrySecRwLtStLgrstUpwdPos_Val
  PA_KeSMSw6sAcsExtSecRwLtStLgrstUpwdDnwdPosMax_Val : Constant  Value=KeSMSw6sAcsExtSecRwLtStLgrstUpwdDnwdPosMax_Val
  PA_KeSMSw6sAcsExtSecRwLtStLgrstUpwdDnwdPosMin_Val : Constant  Value=KeSMSw6sAcsExtSecRwLtStLgrstUpwdDnwdPosMin_Val
  PA_KeSMSw6sAcsExtSecRwLtStLgrstUpwdDnwdPos_Val : Constant  Value=KeSMSw6sAcsExtSecRwLtStLgrstUpwdDnwdPos_Val
  PA_KeSMSw6sRecoveryMdSecRwLtStLgrstUpwdDnwdPosMax_Val : Constant  Value=KeSMSw6sRecoveryMdSecRwLtStLgrstUpwdDnwdPosMax_Val
  PA_KeSMSw6sRecoveryMdSecRwLtStLgrstUpwdDnwdPosMin_Val : Constant  Value=KeSMSw6sRecoveryMdSecRwLtStLgrstUpwdDnwdPosMin_Val
  PA_KeSMSw6sRecoveryMdSecRwLtStLgrstUpwdDnwdPos_Val : Constant  Value=KeSMSw6sRecoveryMdSecRwLtStLgrstUpwdDnwdPos_Val
  PA_KeSMSwAcsEntrySecRwLtStLgrstUpwdPosMax_Val : Constant  Value=KeSMSwAcsEntrySecRwLtStLgrstUpwdPosMax_Val
  PA_KeSMSwAcsEntrySecRwLtStLgrstUpwdPosMin_Val : Constant  Value=KeSMSwAcsEntrySecRwLtStLgrstUpwdPosMin_Val
  PA_KeSMSwAcsEntrySecRwLtStLgrstUpwdPos_Val : Constant  Value=KeSMSwAcsEntrySecRwLtStLgrstUpwdPos_Val
  PA_KeSMSwAcsExtSecRwLtStLgrstUpwdDnwdPosMax_Val : Constant  Value=KeSMSwAcsExtSecRwLtStLgrstUpwdDnwdPosMax_Val
  PA_KeSMSwAcsExtSecRwLtStLgrstUpwdDnwdPosMin_Val : Constant  Value=KeSMSwAcsExtSecRwLtStLgrstUpwdDnwdPosMin_Val
  PA_KeSMSwAcsExtSecRwLtStLgrstUpwdDnwdPos_Val : Constant  Value=KeSMSwAcsExtSecRwLtStLgrstUpwdDnwdPos_Val
  PA_KeSMSwAcsMd56SecRwLtStLgrstUpwdPosMax_Val : Constant  Value=KeSMSwAcsMd56SecRwLtStLgrstUpwdPosMax_Val
  PA_KeSMSwAcsMd56SecRwLtStLgrstUpwdPosMin_Val : Constant  Value=KeSMSwAcsMd56SecRwLtStLgrstUpwdPosMin_Val
  PA_KeSMSwAcsMd56SecRwLtStLgrstUpwdPos_Val : Constant  Value=KeSMSwAcsMd56SecRwLtStLgrstUpwdPos_Val
  PA_KeSMSwAcsMd8SecRwLtStLgrstUpwdDnwdPosMax_Val : Constant  Value=KeSMSwAcsMd8SecRwLtStLgrstUpwdDnwdPosMax_Val
  PA_KeSMSwAcsMd8SecRwLtStLgrstUpwdDnwdPosMin_Val : Constant  Value=KeSMSwAcsMd8SecRwLtStLgrstUpwdDnwdPosMin_Val
  PA_KeSMSwAcsMd8SecRwLtStLgrstUpwdDnwdPos_Val : Constant  Value=KeSMSwAcsMd8SecRwLtStLgrstUpwdDnwdPos_Val
  PA_KeSMSwRecoveryMdSecRwLtStLgrstUpwdDnwdPosMax_Val : Constant  Value=KeSMSwRecoveryMdSecRwLtStLgrstUpwdDnwdPosMax_Val
  PA_KeSMSwRecoveryMdSecRwLtStLgrstUpwdDnwdPosMin_Val : Constant  Value=KeSMSwRecoveryMdSecRwLtStLgrstUpwdDnwdPosMin_Val
  PA_KeSMSwRecoveryMdSecRwLtStLgrstUpwdDnwdPos_Val : Constant  Value=KeSMSwRecoveryMdSecRwLtStLgrstUpwdDnwdPos_Val
  TrgtPosSelc : TrgtPosSelcLib/TrgtPosSelc  SystemSampleTime=-1  VariantActivationTime=update diagram  AllowFlexibleInterface=on  Latency=0  AutoFrameSizeCalculation=off
  TrgtPosSelcNo4sMd : TrgtPosSelcLib/TrgtPosSelcNo4sMd  SystemSampleTime=-1  VariantActivationTime=update diagram  AllowFlexibleInterface=on  Latency=0  AutoFrameSizeCalculation=off
  TrgtPosSelcNo4sMd1 : TrgtPosSelcLib/TrgtPosSelcNo4sMd  Commented=on  SystemSampleTime=-1  VariantActivationTime=update diagram  AllowFlexibleInterface=on  Latency=0  AutoFrameSizeCalculation=off
  TrgtPosSelcNo4sMd2 : TrgtPosSelcLib/TrgtPosSelcNo4sMd  SystemSampleTime=-1  VariantActivationTime=update diagram  AllowFlexibleInterface=on  Latency=0  AutoFrameSizeCalculation=off
  TrgtPosSelcNo4sMd3 : TrgtPosSelcLib/TrgtPosSelcNo4sMd  SystemSampleTime=-1  VariantActivationTime=update diagram  AllowFlexibleInterface=on  Latency=0  AutoFrameSizeCalculation=off
  TrgtPosSelcOnly4sMd{,1..4} (5 alike) : TrgtPosSelcLib/TrgtPosSelcOnly4sMd  Commented=on  SystemSampleTime=-1  VariantActivationTime=update diagram  AllowFlexibleInterface=on  Latency=0  AutoFrameSizeCalculation=off
  EZER2LLgrstUpwdDnwdTrgtPosCalib_TrgtPosArray_write : Outport  VectorParamsAs1DForOutWhenUnconnected=off
  EZQR2LLgrstUpwdDnwdTrgtPosCalib_TrgtPosArray_write : Outport  Port=2  VectorParamsAs1DForOutWhenUnconnected=off
  LgrstCloseLR2LLgrstUpwdDnwdTrgtPosCalib_TrgtPosArray_write : Outport  Port=3  VectorParamsAs1DForOutWhenUnconnected=off
  LgrstOpenLR2LLgrstUpwdDnwdTrgtPosCalib_TrgtPosArray_write : Outport  Port=4  VectorParamsAs1DForOutWhenUnconnected=off
  LyLR2LLgrstUpwdDnwdTrgtPosCalib_TrgtPosArray_write : Outport  Port=5  VectorParamsAs1DForOutWhenUnconnected=off
  RecvLR2LLgrstUpwdDnwdTrgtPosCalib_TrgtPosArray_write : Outport  Port=6  VectorParamsAs1DForOutWhenUnconnected=off
  KeSMSw4SAcsMd22LgrstUpwdDnwdTrgtPosCalib_TrgtPosArray_write : Outport  Port=7  VectorParamsAs1DForOutWhenUnconnected=off
  KeSMSw4SAcsMd26LgrstUpwdDnwdTrgtPosCalib_TrgtPosArray_write : Outport  Port=8  VectorParamsAs1DForOutWhenUnconnected=off
  Md56R2LLgrstUpwdDnwdTrgtPosCalib_TrgtPosArray_write : Outport  Port=9  VectorParamsAs1DForOutWhenUnconnected=off
  Md8R2LLgrstUpwdDnwdTrgtPosCalib_TrgtPosArray_write : Outport  Port=10  VectorParamsAs1DForOutWhenUnconnected=off
  wires:
  PA_KeSMSw6sRecoveryMdSecRwLtStLgrstUpwdDnwdPos_Val/1 -> TrgtPosSelc/6
  [Is6s] -> TrgtPosSelcNo4sMd1/1
  [Is6s] -> TrgtPosSelc/2
  PA_KeSMSw6sAcsExtSecRwLtStLgrstUpwdDnwdPosMin_Val/1 -> TrgtPosSelcNo4sMd1/4
  TrgtPosSelcNo4sMd1/1 -> Data Type Conversion4/1
  PA_KeSMSwAcsExtSecRwLtStLgrstUpwdDnwdPosMax_Val/1 -> TrgtPosSelcNo4sMd1/6
  PA_KeSMSw4SLegrstOpenMdSecRwLtStLgrstUpwdDnwdPosMin_Val/1 -> TrgtPosSelcOnly4sMd2/3
  PA_KeSMSw6sAcsExtSecRwLtStLgrstUpwdDnwdPos_Val/1 -> TrgtPosSelcNo4sMd1/2
  StNumFlg_Is4s_read/1 -> [Is4s], TrgtPosSelc/1
  PA_KeSMSw6sAcsExtSecRwLtStLgrstUpwdDnwdPosMax_Val/1 -> TrgtPosSelcNo4sMd1/3
  PA_KeSMSwAcsExtSecRwLtStLgrstUpwdDnwdPos_Val/1 -> TrgtPosSelcNo4sMd1/5
  PA_KeSMSwAcsExtSecRwLtStLgrstUpwdDnwdPosMin_Val/1 -> TrgtPosSelcNo4sMd1/7
  PA_KeSMSw4sRecoveryMDSecRwLtStLgrstUpwdDnwdPosMax_Val/1 -> TrgtPosSelc/4
  TrgtPosSelcOnly4sMd/1 -> Data Type Conversion8/1
  PA_KeSMSw4sRecoveryMDSecRwLtStLgrstUpwdDnwdPosMin_Val/1 -> TrgtPosSelc/5
  PA_KeSMSw4sRecoveryMDSecRwLtStLgrstUpwdDnwdPos_Val/1 -> TrgtPosSelc/3
  TrgtPosSelcNo4sMd/1 -> Data Type Conversion5/1
  PA_KeSMSw4SLegrstCloseMdSecRwLtStLgrstUpwdDnwdPosMax_Val/1 -> TrgtPosSelcOnly4sMd/2
  PA_KeSMSw6sAcsEntrySecRwLtStLgrstUpwdPosMin_Val/1 -> TrgtPosSelcNo4sMd/4
  PA_KeSMSw4sLyingMDSecRwLtStLgrstUpwdDnwdPosMax_Val/1 -> TrgtPosSelcOnly4sMd1/2
  PA_KeSMSw4SLegrstCloseMdSecRwLtStLgrstUpwdDnwdPosMin_Val/1 -> TrgtPosSelcOnly4sMd/3
  PA_KeSMSw4sLyingMDSecRwLtStLgrstUpwdDnwdPosMin_Val/1 -> TrgtPosSelcOnly4sMd1/3
  PA_KeSMSw6sAcsEntrySecRwLtStLgrstUpwdPosMax_Val/1 -> TrgtPosSelcNo4sMd/3
  PA_KeSMSw6sRecoveryMdSecRwLtStLgrstUpwdDnwdPosMax_Val/1 -> TrgtPosSelc/7
  PA_KeSMSwAcsEntrySecRwLtStLgrstUpwdPosMin_Val/1 -> TrgtPosSelcNo4sMd/7
  PA_KeSMSwAcsEntrySecRwLtStLgrstUpwdPosMax_Val/1 -> TrgtPosSelcNo4sMd/6
  PA_KeSMSwAcsEntrySecRwLtStLgrstUpwdPos_Val/1 -> TrgtPosSelcNo4sMd/5
  PA_KeSMSw4SLegrstOpenMdSecRwLtStLgrstUpwdDnwdPosMax_Val/1 -> TrgtPosSelcOnly4sMd2/2
  TrgtPosSelcOnly4sMd2/1 -> Data Type Conversion7/1
  PA_KeSMSw4SLegrstOpenMdSecRwLtStLgrstUpwdDnwdPos_Val/1 -> TrgtPosSelcOnly4sMd2/1
  PA_KeSMSwRecoveryMdSecRwLtStLgrstUpwdDnwdPos_Val/1 -> TrgtPosSelc/9
  StNumFlg_Is6s_read/1 -> [Is6s], TrgtPosSelcNo4sMd/1
  TrgtPosSelcOnly4sMd1/1 -> Data Type Conversion6/1
  PA_KeSMSw4sLyingMDSecRwLtStLgrstUpwdDnwdPos_Val/1 -> TrgtPosSelcOnly4sMd1/1
  PA_KeSMSw6sRecoveryMdSecRwLtStLgrstUpwdDnwdPosMin_Val/1 -> TrgtPosSelc/8
  PA_KeSMSwRecoveryMdSecRwLtStLgrstUpwdDnwdPosMax_Val/1 -> TrgtPosSelc/10
  PA_KeSMSwRecoveryMdSecRwLtStLgrstUpwdDnwdPosMin_Val/1 -> TrgtPosSelc/11
  PA_KeSMSw6sAcsEntrySecRwLtStLgrstUpwdPos_Val/1 -> TrgtPosSelcNo4sMd/2
  PA_KeSMSw4SLegrstCloseMdSecRwLtStLgrstUpwdDnwdPos_Val/1 -> TrgtPosSelcOnly4sMd/1
  TrgtPosSelc/1 -> Data Type Conversion3/1
  TrgtPosSelcOnly4sMd3/1 -> Data Type Conversion1/1
  TrgtPosSelcOnly4sMd4/1 -> Data Type Conversion/1
  PA_KeSMSw4SAcsMd22SecRwLtStLegrstUpwdDnwdPosMax_Val/1 -> TrgtPosSelcOnly4sMd3/2
  PA_KeSMSw4SAcsMd22SecRwLtStLegrstUpwdDnwdPosMin_Val/1 -> TrgtPosSelcOnly4sMd3/3
  PA_KeSMSw4SAcsMd22SecRwLtStLegrstUpwdDnwdPos_Val/1 -> TrgtPosSelcOnly4sMd3/1
  PA_KeSMSw4SAcsMd26SecRwLtStLegrstUpwdDnwdPosMax_Val/1 -> TrgtPosSelcOnly4sMd4/2
  PA_KeSMSw4SAcsMd26SecRwLtStLegrstUpwdDnwdPosMin_Val/1 -> TrgtPosSelcOnly4sMd4/3
  PA_KeSMSw4SAcsMd26SecRwLtStLegrstUpwdDnwdPos_Val/1 -> TrgtPosSelcOnly4sMd4/1
  Data Type Conversion/1 -> KeSMSw4SAcsMd26LgrstUpwdDnwdTrgtPosCalib_TrgtPosArray_write/1
  Data Type Conversion1/1 -> KeSMSw4SAcsMd22LgrstUpwdDnwdTrgtPosCalib_TrgtPosArray_write/1
  Data Type Conversion3/1 -> RecvLR2LLgrstUpwdDnwdTrgtPosCalib_TrgtPosArray_write/1
  Data Type Conversion4/1 -> EZQR2LLgrstUpwdDnwdTrgtPosCalib_TrgtPosArray_write/1
  Data Type Conversion5/1 -> EZER2LLgrstUpwdDnwdTrgtPosCalib_TrgtPosArray_write/1
  Data Type Conversion6/1 -> LyLR2LLgrstUpwdDnwdTrgtPosCalib_TrgtPosArray_write/1
  Data Type Conversion7/1 -> LgrstOpenLR2LLgrstUpwdDnwdTrgtPosCalib_TrgtPosArray_write/1
  Data Type Conversion8/1 -> LgrstCloseLR2LLgrstUpwdDnwdTrgtPosCalib_TrgtPosArray_write/1
  TrgtPosSelcNo4sMd2/1 -> Data Type Conversion2/1
  Constant/1 -> TrgtPosSelcNo4sMd2/2
  [Is6s] -> TrgtPosSelcNo4sMd2/1
  Constant2/1 -> TrgtPosSelcNo4sMd2/4
  PA_KeSMSwAcsMd8SecRwLtStLgrstUpwdDnwdPosMin_Val/1 -> TrgtPosSelcNo4sMd2/7
  PA_KeSMSwAcsMd8SecRwLtStLgrstUpwdDnwdPosMax_Val/1 -> TrgtPosSelcNo4sMd2/6
  PA_KeSMSwAcsMd8SecRwLtStLgrstUpwdDnwdPos_Val/1 -> TrgtPosSelcNo4sMd2/5
  Constant1/1 -> TrgtPosSelcNo4sMd2/3
  Data Type Conversion2/1 -> Md8R2LLgrstUpwdDnwdTrgtPosCalib_TrgtPosArray_write/1
  TrgtPosSelcNo4sMd3/1 -> Data Type Conversion9/1
  Data Type Conversion9/1 -> Md56R2LLgrstUpwdDnwdTrgtPosCalib_TrgtPosArray_write/1
  [Is6s] -> TrgtPosSelcNo4sMd3/1
  PA_KeSMSw6SAcsMd56SecRwLtStLgrstUpwdPos_Val/1 -> TrgtPosSelcNo4sMd3/2
  PA_KeSMSw6SAcsMd56SecRwLtStLgrstUpwdPosMax_Val/1 -> TrgtPosSelcNo4sMd3/3
  PA_KeSMSw6SAcsMd56SecRwLtStLgrstUpwdPosMin_Val/1 -> TrgtPosSelcNo4sMd3/4
  PA_KeSMSwAcsMd56SecRwLtStLgrstUpwdPosMin_Val/1 -> TrgtPosSelcNo4sMd3/7
  PA_KeSMSwAcsMd56SecRwLtStLgrstUpwdPosMax_Val/1 -> TrgtPosSelcNo4sMd3/6
  PA_KeSMSwAcsMd56SecRwLtStLgrstUpwdPos_Val/1 -> TrgtPosSelcNo4sMd3/5

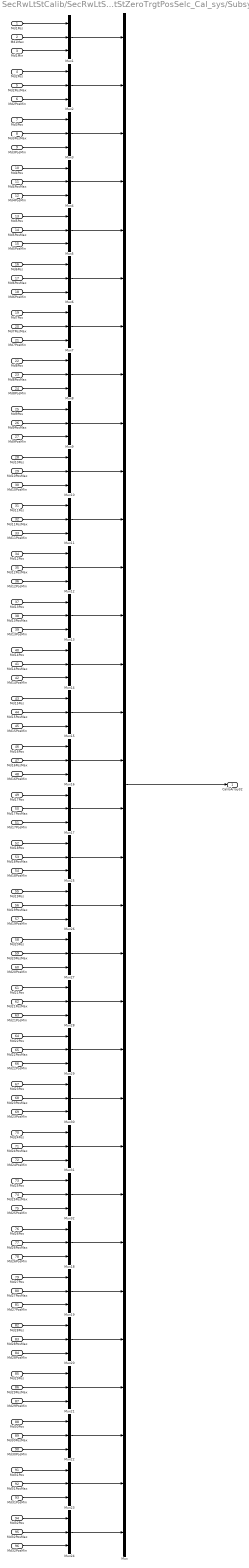
== system SecRwLtStCalib/SecRwLtStZeroTrgtPosSelc_1_Cal_sys/SecRwLtStZeroTrgtPosSelc_Cal_sys/Subsystem ==
  Md1Pos : Inport
  Md1Max : Inport  Port=2
  Md1Min : Inport  Port=3
  Md2Pos : Inport  Port=4
  Md2PosMax : Inport  Port=5
  Md2PosMin : Inport  Port=6
  Md3Pos : Inport  Port=7
  Md3PosMax : Inport  Port=8
  Md3PosMin : Inport  Port=9
  Md4Pos : Inport  Port=10
  Md4PosMax : Inport  Port=11
  Md4PosMin : Inport  Port=12
  Md5Pos : Inport  Port=13
  Md5PosMax : Inport  Port=14
  Md5PosMin : Inport  Port=15
  Md6Pos : Inport  Port=16
  Md6PosMax : Inport  Port=17
  Md6PosMin : Inport  Port=18
  Md7Pos : Inport  Port=19
  Md7PosMax : Inport  Port=20
  Md7PosMin : Inport  Port=21
  Md8Pos : Inport  Port=22
  Md8PosMax : Inport  Port=23
  Md8PosMin : Inport  Port=24
  Md9Pos : Inport  Port=25
  Md9PosMax : Inport  Port=26
  Md9PosMin : Inport  Port=27
  Md10Pos : Inport  Port=28
  Md10PosMax : Inport  Port=29
  Md10PosMin : Inport  Port=30
  Md11Pos : Inport  Port=31
  Md11PosMax : Inport  Port=32
  Md11PosMin : Inport  Port=33
  Md12Pos : Inport  Port=34
  Md12PosMax : Inport  Port=35
  Md12PosMin : Inport  Port=36
  Md13Pos : Inport  Port=37
  Md13PosMax : Inport  Port=38
  Md13PosMin : Inport  Port=39
  Md14Pos : Inport  Port=40
  Md14PosMax : Inport  Port=41
  Md14PosMin : Inport  Port=42
  Md15Pos : Inport  Port=43
  Md15PosMax : Inport  Port=44
  Md15PosMin : Inport  Port=45
  Md16Pos : Inport  Port=46
  Md16PosMax : Inport  Port=47
  Md16PosMin : Inport  Port=48
  Md17Pos : Inport  Port=49
  Md17PosMax : Inport  Port=50
  Md17PosMin : Inport  Port=51
  Md18Pos : Inport  Port=52
  Md18PosMax : Inport  Port=53
  Md18PosMin : Inport  Port=54
  Md19Pos : Inport  Port=55
  Md19PosMax : Inport  Port=56
  Md19PosMin : Inport  Port=57
  Md20Pos : Inport  Port=58
  Md20PosMax : Inport  Port=59
  Md20PosMin : Inport  Port=60
  Md21Pos : Inport  Port=61
  Md21PosMax : Inport  Port=62
  Md21PosMin : Inport  Port=63
  Md22Pos : Inport  Port=64
  Md22PosMax : Inport  Port=65
  Md22PosMin : Inport  Port=66
  Md23Pos : Inport  Port=67
  Md23PosMax : Inport  Port=68
  Md23PosMin : Inport  Port=69
  Md24Pos : Inport  Port=70
  Md24PosMax : Inport  Port=71
  Md24PosMin : Inport  Port=72
  Md25Pos : Inport  Port=73
  Md25PosMax : Inport  Port=74
  Md25PosMin : Inport  Port=75
  Md26Pos : Inport  Port=76
  Md26PosMax : Inport  Port=77
  Md26PosMin : Inport  Port=78
  Md27Pos : Inport  Port=79
  Md27PosMax : Inport  Port=80
  Md27PosMin : Inport  Port=81
  Md28Pos : Inport  Port=82
  Md28PosMax : Inport  Port=83
  Md28PosMin : Inport  Port=84
  Md29Pos : Inport  Port=85
  Md29PosMax : Inport  Port=86
  Md29PosMin : Inport  Port=87
  Md30Pos : Inport  Port=88
  Md30PosMax : Inport  Port=89
  Md30PosMin : Inport  Port=90
  Md31Pos : Inport  Port=91
  Md31PosMax : Inport  Port=92
  Md31PosMin : Inport  Port=93
  Md32Pos : Inport  Port=94
  Md32PosMax : Inport  Port=95
  Md32PosMin : Inport  Port=96
  Mux : Mux  Inputs=32
  Mux{1..32} (32 alike) : Mux  Inputs=3
  CalibArray32 : Outport  VectorParamsAs1DForOutWhenUnconnected=off
  wires:
  Md22PosMax/1 -> Mux29/2
  Md3PosMin/1 -> Mux3/3
  Mux13/1 -> Mux/13
  Md13Pos/1 -> Mux13/1
  Mux30/1 -> Mux/23
  Md2PosMax/1 -> Mux2/2
  Md12PosMin/1 -> Mux12/3
  Md15PosMax/1 -> Mux15/2
  Md17Pos/1 -> Mux17/1
  Mux20/1 -> Mux/28
  Mux27/1 -> Mux/20
  Mux11/1 -> Mux/11
  Mux31/1 -> Mux/24
  Mux24/1 -> Mux/32
  Md8PosMin/1 -> Mux8/3
  Mux7/1 -> Mux/7
  Md20Pos/1 -> Mux27/1
  Mux6/1 -> Mux/6
  Md2PosMin/1 -> Mux2/3
  Md2Pos/1 -> Mux2/1
  Md5Pos/1 -> Mux5/1
  Md4PosMax/1 -> Mux4/2
  Mux25/1 -> Mux/18
  Md5PosMin/1 -> Mux5/3
  Md16PosMin/1 -> Mux16/3
  Md12PosMax/1 -> Mux12/2
  Mux32/1 -> Mux/25
  Md15PosMin/1 -> Mux15/3
  Mux15/1 -> Mux/15
  Mux16/1 -> Mux/16
  Mux21/1 -> Mux/29
  Md27PosMax/1 -> Mux19/2
  Md28Pos/1 -> Mux20/1
  Md13PosMin/1 -> Mux13/3
  Mux29/1 -> Mux/22
  Md8Pos/1 -> Mux8/1
  Mux23/1 -> Mux/31
  Mux22/1 -> Mux/30
  Mux12/1 -> Mux/12
  Md24Pos/1 -> Mux31/1
  Mux9/1 -> Mux/9
  Mux8/1 -> Mux/8
  Md9Pos/1 -> Mux9/1
  Mux3/1 -> Mux/3
  Md6PosMin/1 -> Mux6/3
  Mux17/1 -> Mux/17
  Md6Pos/1 -> Mux6/1
  Mux14/1 -> Mux/14
  Mux1/1 -> Mux/1
  Md10Pos/1 -> Mux10/1
  Md9PosMax/1 -> Mux9/2
  Mux26/1 -> Mux/19
  Mux18/1 -> Mux/26
  Mux28/1 -> Mux/21
  Mux2/1 -> Mux/2
  Mux19/1 -> Mux/27
  Mux10/1 -> Mux/10
  Mux5/1 -> Mux/5
  Md23PosMin/1 -> Mux30/3
  Md4PosMin/1 -> Mux4/3
  Md7PosMin/1 -> Mux7/3
  Md4Pos/1 -> Mux4/1
  Mux4/1 -> Mux/4
  Md13PosMax/1 -> Mux13/2
  Md6PosMax/1 -> Mux6/2
  Md5PosMax/1 -> Mux5/2
  Md14PosMax/1 -> Mux14/2
  Md14PosMin/1 -> Mux14/3
  Md23PosMax/1 -> Mux30/2
  Md1Min/1 -> Mux1/3
  Md8PosMax/1 -> Mux8/2
  Md23Pos/1 -> Mux30/1
  Md1Pos/1 -> Mux1/1
  Md1Max/1 -> Mux1/2
  Md9PosMin/1 -> Mux9/3
  Md7PosMax/1 -> Mux7/2
  Md20PosMin/1 -> Mux27/3
  Md7Pos/1 -> Mux7/1
  Md10PosMax/1 -> Mux10/2
  Md10PosMin/1 -> Mux10/3
  Md15Pos/1 -> Mux15/1
  Md30PosMax/1 -> Mux22/2
  Md11PosMax/1 -> Mux11/2
  Md12Pos/1 -> Mux12/1
  Md11PosMin/1 -> Mux11/3
  Md11Pos/1 -> Mux11/1
  Md14Pos/1 -> Mux14/1
  Md16Pos/1 -> Mux16/1
  Md24PosMin/1 -> Mux31/3
  Md16PosMax/1 -> Mux16/2
  Md32PosMin/1 -> Mux24/3
  Md27Pos/1 -> Mux19/1
  Md32PosMax/1 -> Mux24/2
  Md18Pos/1 -> Mux25/1
  Md19Pos/1 -> Mux26/1
  Md19PosMax/1 -> Mux26/2
  Md21Pos/1 -> Mux28/1
  Md27PosMin/1 -> Mux19/3
  Md26PosMax/1 -> Mux18/2
  Md26PosMin/1 -> Mux18/3
  Md31Pos/1 -> Mux23/1
  Md25Pos/1 -> Mux32/1
  Md28PosMin/1 -> Mux20/3
  Md25PosMin/1 -> Mux32/3
  Md25PosMax/1 -> Mux32/2
  Md17PosMin/1 -> Mux17/3
  Md32Pos/1 -> Mux24/1
  Md24PosMax/1 -> Mux31/2
  Md18PosMax/1 -> Mux25/2
  Md21PosMin/1 -> Mux28/3
  Md30PosMin/1 -> Mux22/3
  Md21PosMax/1 -> Mux28/2
  Md22Pos/1 -> Mux29/1
  Md18PosMin/1 -> Mux25/3
  Md26Pos/1 -> Mux18/1
  Md20PosMax/1 -> Mux27/2
  Md31PosMin/1 -> Mux23/3
  Md29Pos/1 -> Mux21/1
  Md19PosMin/1 -> Mux26/3
  Md29PosMin/1 -> Mux21/3
  Md30Pos/1 -> Mux22/1
  Md17PosMax/1 -> Mux17/2
  Md28PosMax/1 -> Mux20/2
  Md22PosMin/1 -> Mux29/3
  Md31PosMax/1 -> Mux23/2
  Md29PosMax/1 -> Mux21/2
  Mux/1 -> CalibArray32/1
  Md3Pos/1 -> Mux3/1
  Md3PosMax/1 -> Mux3/2
